simulink model "LQR_QRLsim"  (R2013b)
settings: Solver=ode45  StartTime=0.0  StopTime=Tsim_end  MaxStep=.1  RelTol=1e-3
values from neighbouring files (symbols this model uses):
  K = lqr(LQRA,LQRB,LQRQ,LQRR)    [LQRrunfile.m]
  LQRA = [zeros(8) eye(8) ... (first row only)    [LQRrunfile.m]
  LQRB = [zeros(10,4) ... (first row only)    [LQRrunfile.m]
  LQRC = eye(16)    [LQRrunfile.m]
  omega_n1_xL = 2*pi*.4    (= 2.51327412287)    [LQRrunfile.m]    (also in QRLrunfile.m = 25)
  omega_n2_xL = 2*pi*.4    (= 2.51327412287)    [LQRrunfile.m]
undefined symbols (not defined in the file or in its folder): sigbuilder_block, T0
libraries: CF3 x10, simulink x10, simulink_extras x2
settings Model: Creator=Nam  LastModifiedBy=Nam

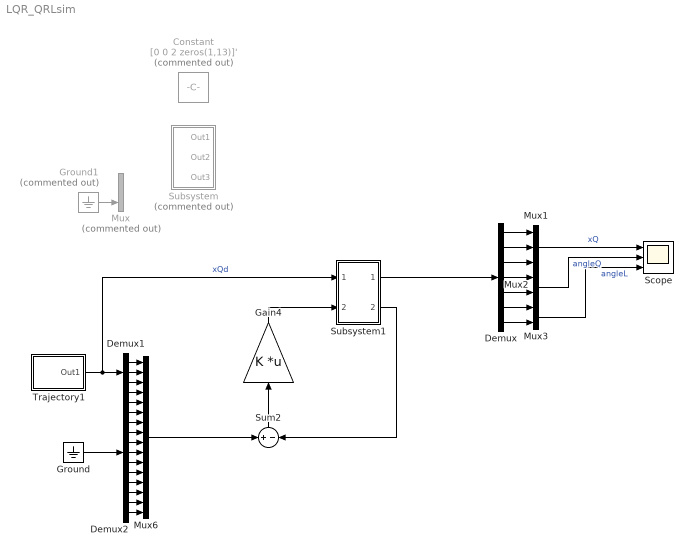
== system LQR_QRLsim ==
  Constant : Constant  Commented=on  Value=[0 0 2 zeros(1,13)]'
  Demux : Demux  Outputs=7
  Demux1 : Demux  Outputs=3
  Demux2 : Demux  Outputs=13
  Gain4 : Gain  Gain=K  Multiplication=Matrix(K*u)
  Ground : Ground
  Ground1 : Ground  Commented=on
  Mux : Mux  Commented=on  Inputs=2
  Mux1 : Mux  Inputs=3
  Mux2 : Mux  Inputs=2
  Mux3 : Mux  Inputs=2
  Mux6 : Mux  Inputs=16
  Scope : Scope  NumInputPorts=3
      settings: YMin=-5~-5~-5  YMax=5~5~5  SaveName=ScopeData9
  Subsystem : Subsystem  Commented=on
  Subsystem1 : Subsystem
  Sum2 : Sum  Inputs=+|-
  Trajectory1 : Subsystem
  wires:
  Sum2/1 -> Gain4/1
  Trajectory1/1(Out1) -> Subsystem1/1(In2), Demux1/1  "xQd"
  Demux1/1 -> Mux6/1
  Demux1/2 -> Mux6/2
  Demux1/3 -> Mux6/3
  Demux2/6 -> Mux6/9
  Demux2/11 -> Mux6/14
  Demux2/7 -> Mux6/10
  Demux2/10 -> Mux6/13
  Demux2/8 -> Mux6/11
  Demux2/12 -> Mux6/15
  Demux2/13 -> Mux6/16
  Demux2/5 -> Mux6/8
  Demux2/9 -> Mux6/12
  Demux2/4 -> Mux6/7
  Demux2/1 -> Mux6/4
  Demux2/2 -> Mux6/5
  Demux2/3 -> Mux6/6
  Ground/1 -> Demux2/1
  Gain4/1 -> Subsystem1/2(In1)
  Subsystem1/2(Out1) -> Sum2/2
  Ground1/1 -> Mux/2
  Mux6/1 -> Sum2/1
  Subsystem1/1(Out2) -> Demux/1
  Demux/2 -> Mux1/2
  Demux/1 -> Mux1/1
  Demux/3 -> Mux1/3
  Demux/4 -> Mux2/1
  Demux/5 -> Mux2/2
  Demux/6 -> Mux3/1
  Demux/7 -> Mux3/2
  Mux1/1 -> Scope/1  "xQ"
  Mux2/1 -> Scope/2  "angleQ"
  Mux3/1 -> Scope/3  "angleL"

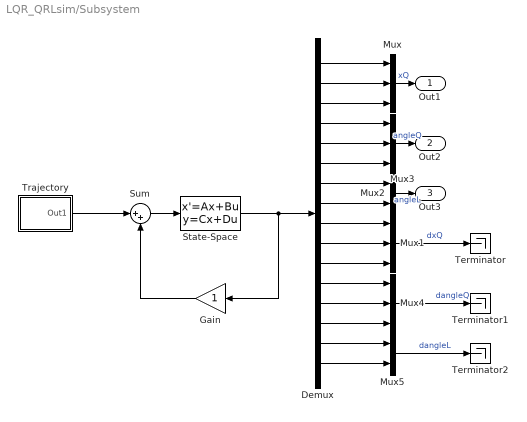
== system LQR_QRLsim/Subsystem ==
  Demux : Demux  Outputs=16
  Gain : Gain
  Mux{,1,3..4} (4 alike) : Mux  Inputs=3
  Mux2 : Mux  Inputs=2
  Mux5 : Mux  Inputs=2
  State-Space : StateSpace  A=LQRA  B=LQRB  C=LQRC  D=0  X0=0
  Sum : Sum  Inputs=|++
  Terminator : Terminator
  Terminator1 : Terminator
  Terminator2 : Terminator
  Trajectory : Subsystem
  Out1 : Outport
  Out2 : Outport  Port=2
  Out3 : Outport  Port=3
  wires:
  Trajectory/1(Out1) -> Sum/1
  Mux/1 -> Out1/1  "xQ"
  Mux3/1 -> Out2/1  "angleQ"
  Mux2/1 -> Out3/1  "angleL"
  Mux1/1 -> Terminator/1  "dxQ"
  Mux4/1 -> Terminator1/1  "dangleQ"
  Gain/1 -> Sum/2
  Demux/13 -> Mux4/2
  Sum/1 -> State-Space/1
  Mux5/1 -> Terminator2/1  "dangleL"
  Demux/16 -> Mux5/2
  Demux/14 -> Mux4/3
  Demux/12 -> Mux4/1
  Demux/15 -> Mux5/1
  Demux/8 -> Mux2/2
  Demux/7 -> Mux2/1
  Demux/10 -> Mux1/2
  Demux/5 -> Mux3/2
  Demux/6 -> Mux3/3
  Demux/9 -> Mux1/1
  Demux/11 -> Mux1/3
  Demux/4 -> Mux3/1
  Demux/1 -> Mux/1
  Demux/2 -> Mux/2
  Demux/3 -> Mux/3
  State-Space/1 -> Demux/1, Gain/1

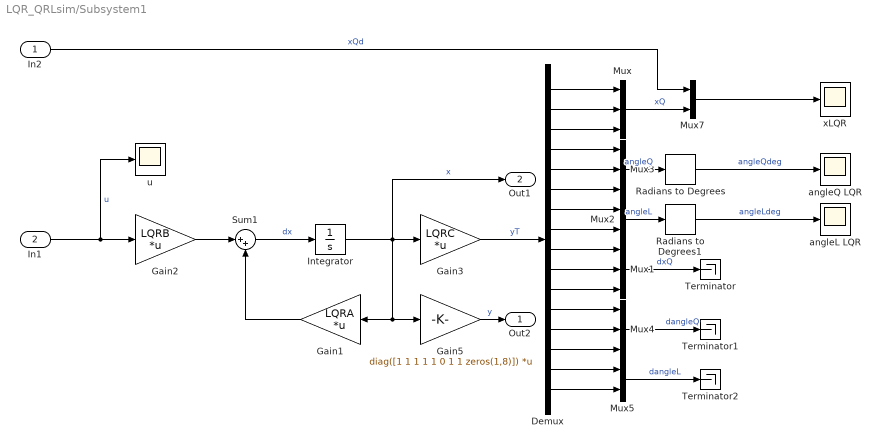
== system LQR_QRLsim/Subsystem1 ==
  In2 : Inport
  In1 : Inport  Port=2
  Demux : Demux  Outputs=16
  Gain1 : Gain  Gain=LQRA  Multiplication=Matrix(K*u)
  Gain2 : Gain  Gain=LQRB  Multiplication=Matrix(K*u)
  Gain3 : Gain  Gain=LQRC  Multiplication=Matrix(K*u)
  Gain5 : Gain  Gain=diag([1 1 1 1 1 0 1 1 zeros(1,8)])  Multiplication=Matrix(K*u)
  Integrator : Integrator
  Mux{,1,3..4} (4 alike) : Mux  Inputs=3
  Mux2 : Mux  Inputs=2
  Mux5 : Mux  Inputs=2
  Mux7 : Mux  Inputs=2
  Radians to Degrees : simulink_extras/Transformations/Radians to Degrees
  Radians to Degrees1 : simulink_extras/Transformations/Radians to Degrees
  Sum1 : Sum  Inputs=|++
  Terminator : Terminator
  Terminator1 : Terminator
  Terminator2 : Terminator
  angleL LQR : Scope
      settings: ShowLegends=on  TimeRange=25  YMin=-40  YMax=40  SaveName=ScopeData5
  angleQ LQR : Scope
      settings: ShowLegends=on  TimeRange=25  YMin=-40  YMax=40  SaveName=ScopeData4
  u : Scope
      settings: ShowLegends=on  SaveName=ScopeData8
  xLQR : Scope
      settings: ShowLegends=on  SaveName=ScopeData3
  Out2 : Outport
  Out1 : Outport  Port=2
  wires:
  Demux/3 -> Mux/3
  Demux/2 -> Mux/2
  Demux/1 -> Mux/1
  Demux/4 -> Mux3/1
  Demux/5 -> Mux3/2
  Demux/6 -> Mux3/3
  Demux/7 -> Mux2/1
  Demux/8 -> Mux2/2
  Demux/10 -> Mux1/2
  Demux/11 -> Mux1/3
  Demux/9 -> Mux1/1
  Demux/12 -> Mux4/1
  Demux/14 -> Mux4/3
  Demux/13 -> Mux4/2
  Demux/15 -> Mux5/1
  Demux/16 -> Mux5/2
  Mux1/1 -> Terminator/1  "dxQ"
  Mux4/1 -> Terminator1/1  "dangleQ"
  Mux5/1 -> Terminator2/1  "dangleL"
  Gain3/1 -> Demux/1  "yT"
  Mux/1 -> Mux7/2  "xQ"
  Mux3/1 -> Radians to Degrees/1  "angleQ"
  Mux2/1 -> Radians to Degrees1/1  "angleL"
  In1/1 -> u/1, Gain2/1  "u"
  Integrator/1 -> Out1/1, Gain3/1, Gain5/1, Gain1/1  "x"
  Sum1/1 -> Integrator/1  "dx"
  Gain1/1 -> Sum1/2
  Gain2/1 -> Sum1/1
  Mux7/1 -> xLQR/1
  Radians to Degrees/1 -> angleQ LQR/1  "angleQdeg"
  Radians to Degrees1/1 -> angleL LQR/1  "angleLdeg"
  In2/1 -> Mux7/1  "xQd"
  Gain5/1 -> Out2/1  "y"

== system LQR_QRLsim/Trajectory1 ==
  Circle : Subsystem  Commented=on
  Manual Switch : ManualSwitch  CurrentSetting=0
  Manual Switch1 : ManualSwitch  CurrentSetting=0
  Path : Subsystem
  Step : Subsystem
  Out1 : Outport
  wires:
  Manual Switch1/1 -> Out1/1  "xLd"
  Manual Switch/1 -> Manual Switch1/2
  Circle/1(Out3) -> Manual Switch1/1
  Path/1(Out3) -> Manual Switch/1
  Step/1(Out2) -> Manual Switch/2

== system LQR_QRLsim/Subsystem/Trajectory ==
  Circle : Subsystem
  Manual Switch : ManualSwitch
  Manual Switch1 : ManualSwitch  CurrentSetting=0
  Path : Subsystem
  Step : Subsystem
  Out1 : Outport
  wires:
  Step/1(Out2) -> Manual Switch/2
  Path/1(Out3) -> Manual Switch/1
  Circle/1(Out3) -> Manual Switch1/1
  Manual Switch/1 -> Manual Switch1/2
  Manual Switch1/1 -> Out1/1  "xLd"

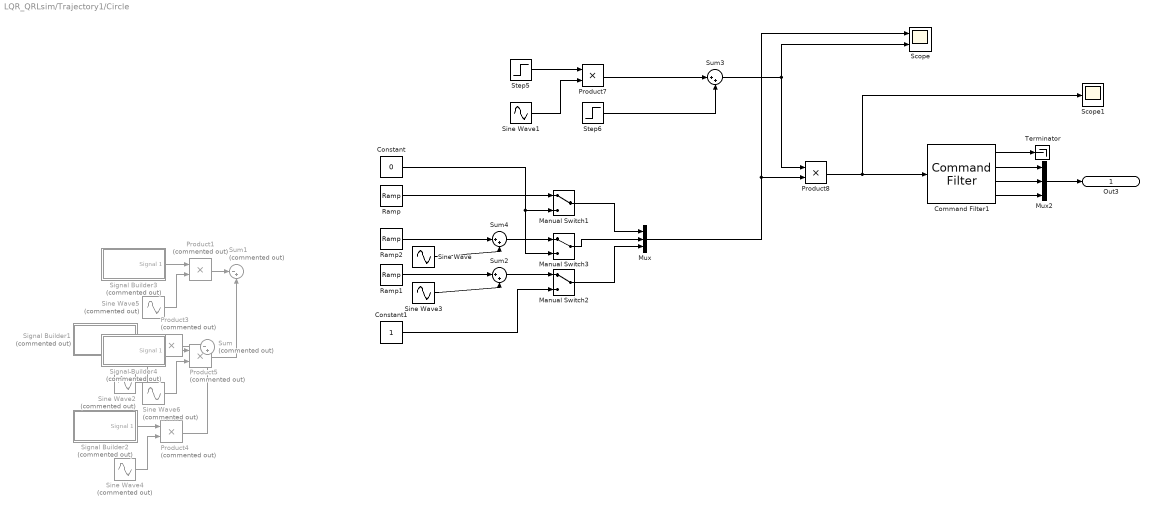
== system LQR_QRLsim/Trajectory1/Circle ==
  Command Filter1 : CF3/Command Filter  Integrator1_init=0  omega_n1=omega_n1_xL  omega_n2=omega_n2_xL  zeta=zeta_xL
  Constant : Constant  Value=0
  Constant1 : Constant
  Manual Switch1 : ManualSwitch
  Manual Switch2 : ManualSwitch
  Manual Switch3 : ManualSwitch
  Mux : Mux  Inputs=3
  Mux2 : Mux  Inputs=3
  Product{1,3..5} (4 alike) : Product  Commented=on
  Product7 : Product
  Product8 : Product
  Ramp : simulink/Sources/Ramp  slope=1/5  start=2  X0=0
  Ramp1 : simulink/Sources/Ramp  slope=0  start=0  X0=0
  Ramp2 : simulink/Sources/Ramp  slope=0  start=0  X0=0
  Scope : Scope  NumInputPorts=2
      settings: ShowLegends=on  YMin=-5~-5  YMax=5~5
  Scope1 : Scope
      settings: ShowLegends=on  YMin=-8  YMax=12  SaveName=ScopeData2
  Signal Builder1 : Subsystem  Tag=STV Subsys  Commented=on  LoadFcn=sigbuilder_block('load');  StartFcn=sigbuilder_block('start');  StopFcn=sigbuilder_block('stop');  ClipboardFcn=sigbuilder_block('clipboard');  mask(Sigbuilder block){}
      mask help: Simulink:masks:SigbuilderBlock_MD
      mask init:
      | if ~strcmp(get_param(bdroot(gcbh),'SimulationStatus'),'stopped') tuvar = sigbuilder_block('maskInit'); end
      settings: CopyFcn=sigbuilder_block('copy');  DeleteFcn=sigbuilder_block('delete');  ModelCloseFcn=sigbuilder_block('modelClose');  PreSaveFcn=sigbuilder_block('preSave');  PauseFcn=sigbuilder_block('pause');  ContinueFcn=sigbuilder_block('continue');  NameChangeFcn=sigbuilder_block('namechange');  OpenFcn=sigbuilder_block('open',[437.25 199.5 550.5 399.75 ]);  CloseFcn=sigbuilder_block('close');
      mask Display: plot(0, 0, 100, 100,[2, 2, 32, 32, 2], [68, 8, 8, 68, 68],[32, 2], [38, 38], [32, 19, 2],[53, 60, 44], [32, 17, 17, 2],[16, 16, 31, 31]);txt = getActiveGroup(gcbh);text(2, 100, txt,'verticalAlignment', 'top');
  Signal Builder2 : Subsystem  Tag=STV Subsys  Commented=on  LoadFcn=sigbuilder_block('load');  StartFcn=sigbuilder_block('start');  StopFcn=sigbuilder_block('stop');  ClipboardFcn=sigbuilder_block('clipboard');  mask(Sigbuilder block){}
      mask help: Simulink:masks:SigbuilderBlock_MD
      mask init:
      | if ~strcmp(get_param(bdroot(gcbh),'SimulationStatus'),'stopped') tuvar = sigbuilder_block('maskInit'); end
      settings: CopyFcn=sigbuilder_block('copy');  DeleteFcn=sigbuilder_block('delete');  ModelCloseFcn=sigbuilder_block('modelClose');  PreSaveFcn=sigbuilder_block('preSave');  PauseFcn=sigbuilder_block('pause');  ContinueFcn=sigbuilder_block('continue');  NameChangeFcn=sigbuilder_block('namechange');  OpenFcn=sigbuilder_block('open',[403.5 199.5 550.5 395.25 ]);  CloseFcn=sigbuilder_block('close');
      mask Display: plot(0, 0, 100, 100,[2, 2, 32, 32, 2], [68, 8, 8, 68, 68],[32, 2], [38, 38], [32, 19, 2],[53, 60, 44], [32, 17, 17, 2],[16, 16, 31, 31]);txt = getActiveGroup(gcbh);text(2, 100, txt,'verticalAlignment', 'top');
  Signal Builder3 : Subsystem  Tag=STV Subsys  Commented=on  LoadFcn=sigbuilder_block('load');  StartFcn=sigbuilder_block('start');  StopFcn=sigbuilder_block('stop');  ClipboardFcn=sigbuilder_block('clipboard');  mask(Sigbuilder block){}
      mask help: Simulink:masks:SigbuilderBlock_MD
      mask init:
      | if ~strcmp(get_param(bdroot(gcbh),'SimulationStatus'),'stopped') tuvar = sigbuilder_block('maskInit'); end
      settings: CopyFcn=sigbuilder_block('copy');  DeleteFcn=sigbuilder_block('delete');  ModelCloseFcn=sigbuilder_block('modelClose');  PreSaveFcn=sigbuilder_block('preSave');  PauseFcn=sigbuilder_block('pause');  ContinueFcn=sigbuilder_block('continue');  NameChangeFcn=sigbuilder_block('namechange');  OpenFcn=sigbuilder_block('open',[437.25 199.5 550.5 399.75 ]);  CloseFcn=sigbuilder_block('close');
      mask Display: plot(0, 0, 100, 100,[2, 2, 32, 32, 2], [68, 8, 8, 68, 68],[32, 2], [38, 38], [32, 19, 2],[53, 60, 44], [32, 17, 17, 2],[16, 16, 31, 31]);txt = getActiveGroup(gcbh);text(2, 100, txt,'verticalAlignment', 'top');
  Signal Builder4 : Subsystem  Tag=STV Subsys  Commented=on  LoadFcn=sigbuilder_block('load');  StartFcn=sigbuilder_block('start');  StopFcn=sigbuilder_block('stop');  ClipboardFcn=sigbuilder_block('clipboard');  mask(Sigbuilder block){}
      mask help: Simulink:masks:SigbuilderBlock_MD
      mask init:
      | if ~strcmp(get_param(bdroot(gcbh),'SimulationStatus'),'stopped') tuvar = sigbuilder_block('maskInit'); end
      settings: CopyFcn=sigbuilder_block('copy');  DeleteFcn=sigbuilder_block('delete');  ModelCloseFcn=sigbuilder_block('modelClose');  PreSaveFcn=sigbuilder_block('preSave');  PauseFcn=sigbuilder_block('pause');  ContinueFcn=sigbuilder_block('continue');  NameChangeFcn=sigbuilder_block('namechange');  OpenFcn=sigbuilder_block('open',[403.5 199.5 550.5 395.25 ]);  CloseFcn=sigbuilder_block('close');
      mask Display: plot(0, 0, 100, 100,[2, 2, 32, 32, 2], [68, 8, 8, 68, 68],[32, 2], [38, 38], [32, 19, 2],[53, 60, 44], [32, 17, 17, 2],[16, 16, 31, 31]);txt = getActiveGroup(gcbh);text(2, 100, txt,'verticalAlignment', 'top');
  Sine Wave : Sin  Amplitude=2.75  Frequency=2*pi/T0  Phase=-pi/2  SampleTime=0
  Sine Wave1 : Sin  Amplitude=0.5  Bias=0.5  Frequency=pi/(T0/2)  Phase=pi*1.5  SampleTime=0
  Sine Wave{2,4..6} (4 alike) : Sin  Commented=on  Amplitude=3  Frequency=2*pi/2.5  SampleTime=0
  Sine Wave3 : Sin  Frequency=2*pi/T0  SampleTime=0
  Step5 : Step  Time=(T0/2)  Before=1  After=0  SampleTime=0
  Step6 : Step  Time=(T0/2)  SampleTime=0
  Sum : Sum  Commented=on  Inputs=|-+
  Sum1 : Sum  Commented=on  Inputs=|-+
  Sum2 : Sum  Inputs=|++
  Sum3 : Sum  Inputs=|++
  Sum4 : Sum  Inputs=|++
  Terminator : Terminator
  Out3 : Outport
  wires:
  Constant/1 -> Manual Switch1/2, Manual Switch3/2
  Sine Wave3/1 -> Sum2/2
  Signal Builder1/1(Signal 1) -> Product3/1
  Sine Wave2/1 -> Product3/2
  Product3/1 -> Sum/1
  Signal Builder2/1(Signal 1) -> Product4/1
  Sine Wave4/1 -> Product4/2
  Product4/1 -> Sum/2
  Manual Switch3/1 -> Mux/2
  Manual Switch2/1 -> Mux/3
  Manual Switch1/1 -> Mux/1
  Mux/1 -> Product8/2, Scope/1
  Sine Wave1/1 -> Product7/2
  Step5/1 -> Product7/1
  Step6/1 -> Sum3/2
  Sum3/1 -> Product8/1, Scope/2
  Constant1/1 -> Manual Switch2/2
  Product7/1 -> Sum3/1
  Product8/1 -> Scope1/1, Command Filter1/1
  Signal Builder3/1(Signal 1) -> Product1/1
  Sine Wave5/1 -> Product1/2
  Product1/1 -> Sum1/1
  Signal Builder4/1(Signal 1) -> Product5/1
  Sine Wave6/1 -> Product5/2
  Product5/1 -> Sum1/2
  Ramp1/1 -> Sum2/1
  Ramp2/1 -> Sum4/1
  Sum4/1 -> Manual Switch3/1
  Sine Wave/1 -> Sum4/2
  Ramp/1 -> Manual Switch1/1
  Sum2/1 -> Manual Switch2/1
  Command Filter1/1 -> Terminator/1
  Command Filter1/3 -> Mux2/2
  Command Filter1/2 -> Mux2/1
  Command Filter1/4 -> Mux2/3
  Mux2/1 -> Out3/1

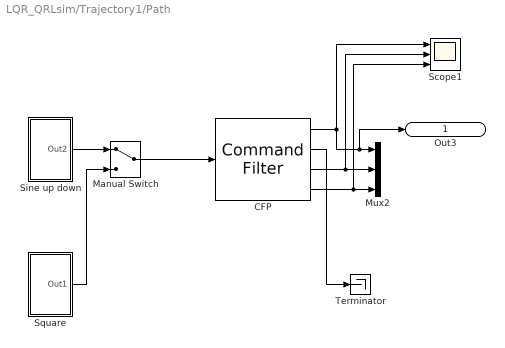
== system LQR_QRLsim/Trajectory1/Path ==
  CFP : CF3/Command Filter  Integrator1_init=0  omega_n1=omega_n1_xL*100  omega_n2=omega_n2_xL*50  zeta=zeta_xL
  Manual Switch : ManualSwitch
  Mux2 : Mux  Inputs=3
  Scope1 : Scope  NumInputPorts=3
      settings: TimeRange=25  YMin=-0.5~-0.8~-1.5  YMax=3.5~0.8~1.5  SaveName=ScopeData6
  Sine up down : Subsystem
  Square : Subsystem
  Terminator : Terminator
  Out3 : Outport
  wires:
  CFP/4 -> Scope1/3, Mux2/3
  CFP/3 -> Scope1/2, Mux2/2
  Manual Switch/1 -> CFP/1
  Square/1(Out1) -> Manual Switch/2
  Sine up down/1(Out2) -> Manual Switch/1
  CFP/1 -> Scope1/1, Out3/1, Mux2/1
  CFP/2 -> Terminator/1

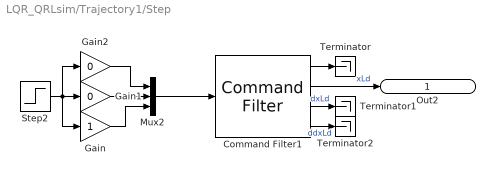
== system LQR_QRLsim/Trajectory1/Step ==
  Command Filter1 : CF3/Command Filter  Integrator1_init=0  omega_n1=2*pi*.75  omega_n2=2*pi*.75  zeta=.975
  Gain : Gain
  Gain1 : Gain  Gain=0
  Gain2 : Gain  Gain=0
  Mux2 : Mux  Inputs=3
  Step2 : Step  SampleTime=0
  Terminator : Terminator
  Terminator1 : Terminator
  Terminator2 : Terminator
  Out2 : Outport
  wires:
  Step2/1 -> Gain2/1, Gain/1, Gain1/1
  Mux2/1 -> Command Filter1/1
  Gain/1 -> Mux2/3
  Gain1/1 -> Mux2/2
  Gain2/1 -> Mux2/1
  Command Filter1/1 -> Terminator/1
  Command Filter1/2 -> Out2/1  "xLd"
  Command Filter1/3 -> Terminator1/1  "dxLd"
  Command Filter1/4 -> Terminator2/1  "ddxLd"

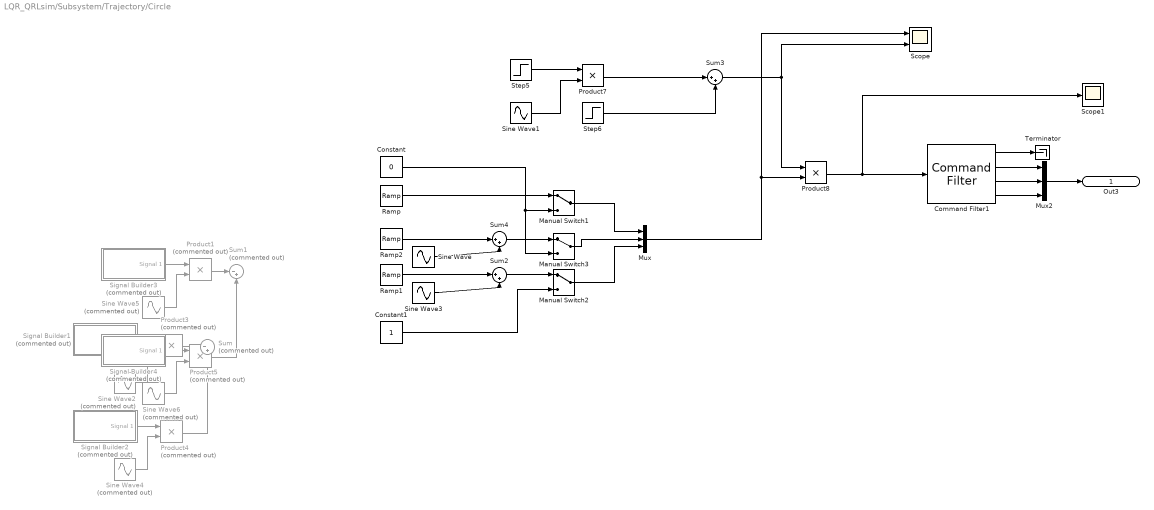
== system LQR_QRLsim/Subsystem/Trajectory/Circle ==
  Command Filter1 : CF3/Command Filter  Integrator1_init=0  omega_n1=omega_n1_xL  omega_n2=omega_n2_xL  zeta=zeta_xL
  Constant : Constant  Value=0
  Constant1 : Constant
  Manual Switch1 : ManualSwitch
  Manual Switch2 : ManualSwitch
  Manual Switch3 : ManualSwitch
  Mux : Mux  Inputs=3
  Mux2 : Mux  Inputs=3
  Product{1,3..5} (4 alike) : Product  Commented=on
  Product7 : Product
  Product8 : Product
  Ramp : simulink/Sources/Ramp  slope=1/5  start=2  X0=0
  Ramp1 : simulink/Sources/Ramp  slope=0  start=0  X0=0
  Ramp2 : simulink/Sources/Ramp  slope=0  start=0  X0=0
  Scope : Scope  NumInputPorts=2
      settings: ShowLegends=on  YMin=-5~-5  YMax=5~5
  Scope1 : Scope
      settings: ShowLegends=on  YMin=-8  YMax=12  SaveName=ScopeData2
  Signal Builder1 : Subsystem  Tag=STV Subsys  Commented=on  LoadFcn=sigbuilder_block('load');  StartFcn=sigbuilder_block('start');  StopFcn=sigbuilder_block('stop');  ClipboardFcn=sigbuilder_block('clipboard');  mask(Sigbuilder block){}
      mask help: Simulink:masks:SigbuilderBlock_MD
      mask init:
      | if ~strcmp(get_param(bdroot(gcbh),'SimulationStatus'),'stopped') tuvar = sigbuilder_block('maskInit'); end
      settings: CopyFcn=sigbuilder_block('copy');  DeleteFcn=sigbuilder_block('delete');  ModelCloseFcn=sigbuilder_block('modelClose');  PreSaveFcn=sigbuilder_block('preSave');  PauseFcn=sigbuilder_block('pause');  ContinueFcn=sigbuilder_block('continue');  NameChangeFcn=sigbuilder_block('namechange');  OpenFcn=sigbuilder_block('open',[437.25 199.5 550.5 399.75 ]);  CloseFcn=sigbuilder_block('close');
      mask Display: plot(0, 0, 100, 100,[2, 2, 32, 32, 2], [68, 8, 8, 68, 68],[32, 2], [38, 38], [32, 19, 2],[53, 60, 44], [32, 17, 17, 2],[16, 16, 31, 31]);txt = getActiveGroup(gcbh);text(2, 100, txt,'verticalAlignment', 'top');
  Signal Builder2 : Subsystem  Tag=STV Subsys  Commented=on  LoadFcn=sigbuilder_block('load');  StartFcn=sigbuilder_block('start');  StopFcn=sigbuilder_block('stop');  ClipboardFcn=sigbuilder_block('clipboard');  mask(Sigbuilder block){}
      mask help: Simulink:masks:SigbuilderBlock_MD
      mask init:
      | if ~strcmp(get_param(bdroot(gcbh),'SimulationStatus'),'stopped') tuvar = sigbuilder_block('maskInit'); end
      settings: CopyFcn=sigbuilder_block('copy');  DeleteFcn=sigbuilder_block('delete');  ModelCloseFcn=sigbuilder_block('modelClose');  PreSaveFcn=sigbuilder_block('preSave');  PauseFcn=sigbuilder_block('pause');  ContinueFcn=sigbuilder_block('continue');  NameChangeFcn=sigbuilder_block('namechange');  OpenFcn=sigbuilder_block('open',[403.5 199.5 550.5 395.25 ]);  CloseFcn=sigbuilder_block('close');
      mask Display: plot(0, 0, 100, 100,[2, 2, 32, 32, 2], [68, 8, 8, 68, 68],[32, 2], [38, 38], [32, 19, 2],[53, 60, 44], [32, 17, 17, 2],[16, 16, 31, 31]);txt = getActiveGroup(gcbh);text(2, 100, txt,'verticalAlignment', 'top');
  Signal Builder3 : Subsystem  Tag=STV Subsys  Commented=on  LoadFcn=sigbuilder_block('load');  StartFcn=sigbuilder_block('start');  StopFcn=sigbuilder_block('stop');  ClipboardFcn=sigbuilder_block('clipboard');  mask(Sigbuilder block){}
      mask help: Simulink:masks:SigbuilderBlock_MD
      mask init:
      | if ~strcmp(get_param(bdroot(gcbh),'SimulationStatus'),'stopped') tuvar = sigbuilder_block('maskInit'); end
      settings: CopyFcn=sigbuilder_block('copy');  DeleteFcn=sigbuilder_block('delete');  ModelCloseFcn=sigbuilder_block('modelClose');  PreSaveFcn=sigbuilder_block('preSave');  PauseFcn=sigbuilder_block('pause');  ContinueFcn=sigbuilder_block('continue');  NameChangeFcn=sigbuilder_block('namechange');  OpenFcn=sigbuilder_block('open',[437.25 199.5 550.5 399.75 ]);  CloseFcn=sigbuilder_block('close');
      mask Display: plot(0, 0, 100, 100,[2, 2, 32, 32, 2], [68, 8, 8, 68, 68],[32, 2], [38, 38], [32, 19, 2],[53, 60, 44], [32, 17, 17, 2],[16, 16, 31, 31]);txt = getActiveGroup(gcbh);text(2, 100, txt,'verticalAlignment', 'top');
  Signal Builder4 : Subsystem  Tag=STV Subsys  Commented=on  LoadFcn=sigbuilder_block('load');  StartFcn=sigbuilder_block('start');  StopFcn=sigbuilder_block('stop');  ClipboardFcn=sigbuilder_block('clipboard');  mask(Sigbuilder block){}
      mask help: Simulink:masks:SigbuilderBlock_MD
      mask init:
      | if ~strcmp(get_param(bdroot(gcbh),'SimulationStatus'),'stopped') tuvar = sigbuilder_block('maskInit'); end
      settings: CopyFcn=sigbuilder_block('copy');  DeleteFcn=sigbuilder_block('delete');  ModelCloseFcn=sigbuilder_block('modelClose');  PreSaveFcn=sigbuilder_block('preSave');  PauseFcn=sigbuilder_block('pause');  ContinueFcn=sigbuilder_block('continue');  NameChangeFcn=sigbuilder_block('namechange');  OpenFcn=sigbuilder_block('open',[403.5 199.5 550.5 395.25 ]);  CloseFcn=sigbuilder_block('close');
      mask Display: plot(0, 0, 100, 100,[2, 2, 32, 32, 2], [68, 8, 8, 68, 68],[32, 2], [38, 38], [32, 19, 2],[53, 60, 44], [32, 17, 17, 2],[16, 16, 31, 31]);txt = getActiveGroup(gcbh);text(2, 100, txt,'verticalAlignment', 'top');
  Sine Wave : Sin  Amplitude=2.75  Frequency=2*pi/T0  Phase=-pi/2  SampleTime=0
  Sine Wave1 : Sin  Amplitude=0.5  Bias=0.5  Frequency=pi/(T0/2)  Phase=pi*1.5  SampleTime=0
  Sine Wave{2,4..6} (4 alike) : Sin  Commented=on  Amplitude=3  Frequency=2*pi/2.5  SampleTime=0
  Sine Wave3 : Sin  Frequency=2*pi/T0  SampleTime=0
  Step5 : Step  Time=(T0/2)  Before=1  After=0  SampleTime=0
  Step6 : Step  Time=(T0/2)  SampleTime=0
  Sum : Sum  Commented=on  Inputs=|-+
  Sum1 : Sum  Commented=on  Inputs=|-+
  Sum2 : Sum  Inputs=|++
  Sum3 : Sum  Inputs=|++
  Sum4 : Sum  Inputs=|++
  Terminator : Terminator
  Out3 : Outport
  wires:
  Mux2/1 -> Out3/1
  Command Filter1/4 -> Mux2/3
  Command Filter1/2 -> Mux2/1
  Command Filter1/3 -> Mux2/2
  Command Filter1/1 -> Terminator/1
  Sum2/1 -> Manual Switch2/1
  Ramp/1 -> Manual Switch1/1
  Sine Wave/1 -> Sum4/2
  Sum4/1 -> Manual Switch3/1
  Ramp2/1 -> Sum4/1
  Ramp1/1 -> Sum2/1
  Product5/1 -> Sum1/2
  Sine Wave6/1 -> Product5/2
  Signal Builder4/1(Signal 1) -> Product5/1
  Product1/1 -> Sum1/1
  Sine Wave5/1 -> Product1/2
  Signal Builder3/1(Signal 1) -> Product1/1
  Product8/1 -> Command Filter1/1, Scope1/1
  Product7/1 -> Sum3/1
  Constant1/1 -> Manual Switch2/2
  Sum3/1 -> Scope/2, Product8/1
  Step6/1 -> Sum3/2
  Step5/1 -> Product7/1
  Sine Wave1/1 -> Product7/2
  Mux/1 -> Scope/1, Product8/2
  Manual Switch1/1 -> Mux/1
  Manual Switch2/1 -> Mux/3
  Manual Switch3/1 -> Mux/2
  Product4/1 -> Sum/2
  Sine Wave4/1 -> Product4/2
  Signal Builder2/1(Signal 1) -> Product4/1
  Product3/1 -> Sum/1
  Sine Wave2/1 -> Product3/2
  Signal Builder1/1(Signal 1) -> Product3/1
  Sine Wave3/1 -> Sum2/2
  Constant/1 -> Manual Switch3/2, Manual Switch1/2

== system LQR_QRLsim/Subsystem/Trajectory/Path ==
  CFP : CF3/Command Filter  Integrator1_init=0  omega_n1=omega_n1_xL*100  omega_n2=omega_n2_xL*50  zeta=zeta_xL
  Manual Switch : ManualSwitch  CurrentSetting=0
  Mux2 : Mux  Inputs=3
  Scope1 : Scope  NumInputPorts=3
      settings: TimeRange=25  YMin=-0.5~-0.8~-1.5  YMax=3.5~0.8~1.5  SaveName=ScopeData6
  Sine up down : Subsystem
  Square : Subsystem
  Terminator : Terminator
  Out3 : Outport
  wires:
  CFP/2 -> Terminator/1
  CFP/1 -> Mux2/1, Scope1/1
  Sine up down/1(Out2) -> Manual Switch/1
  Mux2/1 -> Out3/1
  Square/1(Out1) -> Manual Switch/2
  Manual Switch/1 -> CFP/1
  CFP/3 -> Mux2/2, Scope1/2
  CFP/4 -> Mux2/3, Scope1/3

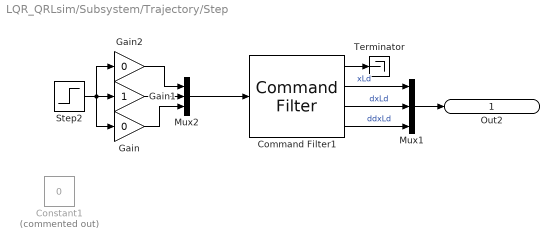
== system LQR_QRLsim/Subsystem/Trajectory/Step ==
  Command Filter1 : CF3/Command Filter  Integrator1_init=0  omega_n1=2*pi*.75  omega_n2=2*pi*.75  zeta=.975
  Constant1 : Constant  Commented=on  Value=0
  Gain : Gain  Gain=0
  Gain1 : Gain
  Gain2 : Gain  Gain=0
  Mux1 : Mux  Inputs=3
  Mux2 : Mux  Inputs=3
  Step2 : Step  SampleTime=0
  Terminator : Terminator
  Out2 : Outport
  wires:
  Mux1/1 -> Out2/1
  Command Filter1/3 -> Mux1/2  "dxLd"
  Command Filter1/2 -> Mux1/1  "xLd"
  Command Filter1/4 -> Mux1/3  "ddxLd"
  Command Filter1/1 -> Terminator/1
  Gain2/1 -> Mux2/1
  Gain1/1 -> Mux2/2
  Gain/1 -> Mux2/3
  Mux2/1 -> Command Filter1/1
  Step2/1 -> Gain1/1, Gain/1, Gain2/1

== system LQR_QRLsim/Trajectory1/Circle/Signal Builder1 ==
  Demux : Demux  Tag=STV Demux  Outputs=1
  FromWs : FromWorkspace  Tag=STV FromWs  VariableName=tuvar  SampleTime=0
      SigBuilderData=|
      | common.afterFinalStr = 'Extrapolate'
      | common.sampleTime = 0
      | dataSet.timeRange = [0 10]
      | dataSet.name = 'Group 1'
      | sbobj.Groups.Name = 'Group 1'
      | sbobj.Groups.Signals.Name = 'Signal 1'
      | sbobj.Groups.Signals.XData = [0 2.5 2.5 10]
      | sbobj.Groups.Signals.YData = [1 1 0 0]
  Signal 1 : Outport  Tag=STV Outport
  wires:
  Demux/1 -> Signal 1/1
  FromWs/1 -> Demux/1

== system LQR_QRLsim/Trajectory1/Circle/Signal Builder2 ==
  Demux : Demux  Tag=STV Demux  Outputs=1
  FromWs : FromWorkspace  Tag=STV FromWs  VariableName=tuvar  SampleTime=0
      SigBuilderData=|
      | common.afterFinalStr = 'Extrapolate'
      | common.sampleTime = 0
      | dataSet.timeRange = [0 10]
      | dataSet.name = 'Group 1'
      | sbobj.Groups.Name = 'Group 1'
      | sbobj.Groups.Signals.Name = 'Signal 1'
      | sbobj.Groups.Signals.XData = [0 2.5 2.5 5 5 10]
      | sbobj.Groups.Signals.YData = [0 0 1 1 0 0]
  Signal 1 : Outport  Tag=STV Outport
  wires:
  Demux/1 -> Signal 1/1
  FromWs/1 -> Demux/1

== system LQR_QRLsim/Trajectory1/Circle/Signal Builder3 ==
  Demux : Demux  Tag=STV Demux  Outputs=1
  FromWs : FromWorkspace  Tag=STV FromWs  VariableName=tuvar  SampleTime=0
      SigBuilderData=|
      | common.afterFinalStr = 'Extrapolate'
      | common.sampleTime = 0
      | dataSet.timeRange = [0 10]
      | dataSet.name = 'Group 1'
      | sbobj.Groups.Name = 'Group 1'
      | sbobj.Groups.Signals.Name = 'Signal 1'
      | sbobj.Groups.Signals.XData = [0 2.5 2.5 10]
      | sbobj.Groups.Signals.YData = [1 1 0 0]
  Signal 1 : Outport  Tag=STV Outport
  wires:
  FromWs/1 -> Demux/1
  Demux/1 -> Signal 1/1

== system LQR_QRLsim/Trajectory1/Circle/Signal Builder4 ==
  Demux : Demux  Tag=STV Demux  Outputs=1
  FromWs : FromWorkspace  Tag=STV FromWs  VariableName=tuvar  SampleTime=0
      SigBuilderData=|
      | common.afterFinalStr = 'Extrapolate'
      | common.sampleTime = 0
      | dataSet.timeRange = [0 10]
      | dataSet.name = 'Group 1'
      | sbobj.Groups.Name = 'Group 1'
      | sbobj.Groups.Signals.Name = 'Signal 1'
      | sbobj.Groups.Signals.XData = [0 2.5 2.5 5 5 10]
      | sbobj.Groups.Signals.YData = [0 0 1 1 0 0]
  Signal 1 : Outport  Tag=STV Outport
  wires:
  FromWs/1 -> Demux/1
  Demux/1 -> Signal 1/1

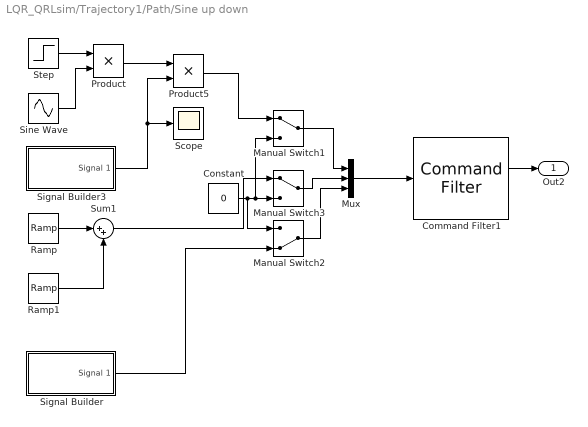
== system LQR_QRLsim/Trajectory1/Path/Sine up down ==
  Command Filter1 : CF3/Command Filter  Integrator1_init=0  omega_n1=omega_n1_xL  omega_n2=omega_n2_xL  zeta=zeta_xL
  Constant : Constant  Value=0
  Manual Switch1 : ManualSwitch
  Manual Switch2 : ManualSwitch  CurrentSetting=0
  Manual Switch3 : ManualSwitch
  Mux : Mux  Inputs=3
  Product : Product
  Product5 : Product
  Ramp : simulink/Sources/Ramp  slope=1/2  start=0  X0=0
  Ramp1 : simulink/Sources/Ramp  slope=-1/2  start=14  X0=0
  Scope : Scope
  Signal Builder : Subsystem  Tag=STV Subsys  LoadFcn=sigbuilder_block('load');  StartFcn=sigbuilder_block('start');  StopFcn=sigbuilder_block('stop');  ClipboardFcn=sigbuilder_block('clipboard');  mask(Sigbuilder block){}
      mask help: Simulink:masks:SigbuilderBlock_MD
      mask init:
      | if ~strcmp(get_param(bdroot(gcbh),'SimulationStatus'),'stopped') tuvar = sigbuilder_block('maskInit'); end
      settings: CopyFcn=sigbuilder_block('copy');  DeleteFcn=sigbuilder_block('delete');  ModelCloseFcn=sigbuilder_block('modelClose');  PreSaveFcn=sigbuilder_block('preSave');  PauseFcn=sigbuilder_block('pause');  ContinueFcn=sigbuilder_block('continue');  NameChangeFcn=sigbuilder_block('namechange');  OpenFcn=sigbuilder_block('open',[611.25 186.75 750 399.75 ]);  CloseFcn=sigbuilder_block('close');
      mask Display: plot(0, 0, 100, 100,[2, 2, 32, 32, 2], [68, 8, 8, 68, 68],[32, 2], [38, 38], [32, 19, 2],[53, 60, 44], [32, 17, 17, 2],[16, 16, 31, 31]);txt = getActiveGroup(gcbh);text(2, 100, txt,'verticalAlignment', 'top');
  Signal Builder3 : Subsystem  Tag=STV Subsys  LoadFcn=sigbuilder_block('load');  StartFcn=sigbuilder_block('start');  StopFcn=sigbuilder_block('stop');  ClipboardFcn=sigbuilder_block('clipboard');  mask(Sigbuilder block){}
      mask help: Simulink:masks:SigbuilderBlock_MD
      mask init:
      | if ~strcmp(get_param(bdroot(gcbh),'SimulationStatus'),'stopped') tuvar = sigbuilder_block('maskInit'); end
      settings: CopyFcn=sigbuilder_block('copy');  DeleteFcn=sigbuilder_block('delete');  ModelCloseFcn=sigbuilder_block('modelClose');  PreSaveFcn=sigbuilder_block('preSave');  PauseFcn=sigbuilder_block('pause');  ContinueFcn=sigbuilder_block('continue');  NameChangeFcn=sigbuilder_block('namechange');  OpenFcn=sigbuilder_block('open',[87.75 213.75 999 399.75 ]);  CloseFcn=sigbuilder_block('close');
      mask Display: plot(0, 0, 100, 100,[2, 2, 32, 32, 2], [68, 8, 8, 68, 68],[32, 2], [38, 38], [32, 19, 2],[53, 60, 44], [32, 17, 17, 2],[16, 16, 31, 31]);txt = getActiveGroup(gcbh);text(2, 100, txt,'verticalAlignment', 'top');
  Sine Wave : Sin  Amplitude=3  Frequency=2*pi/2.5  SampleTime=0
  Step : Step  Time=0  SampleTime=0
  Sum1 : Sum  Inputs=|++
  Out2 : Outport
  wires:
  Mux/1 -> Command Filter1/1
  Constant/1 -> Manual Switch3/2, Manual Switch1/2, Manual Switch2/1
  Manual Switch1/1 -> Mux/1
  Manual Switch2/1 -> Mux/3
  Ramp/1 -> Sum1/1
  Manual Switch3/1 -> Mux/2
  Step/1 -> Product/1
  Sine Wave/1 -> Product/2
  Product/1 -> Product5/1
  Product5/1 -> Manual Switch1/1
  Signal Builder3/1(Signal 1) -> Scope/1, Product5/2
  Ramp1/1 -> Sum1/2
  Sum1/1 -> Manual Switch3/1
  Signal Builder/1(Signal 1) -> Manual Switch2/2
  Command Filter1/2 -> Out2/1

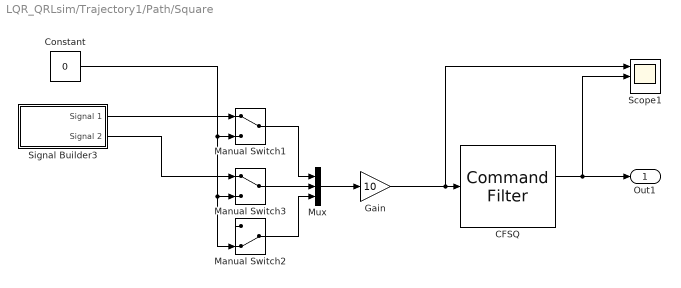
== system LQR_QRLsim/Trajectory1/Path/Square ==
  CFSQ : CF3/Command Filter  Integrator1_init=0  omega_n1=2*pi*1.2*0.5  omega_n2=2*pi*1*.5  zeta=zeta_xL
  Constant : Constant  Value=0
  Gain : Gain  Gain=10
  Manual Switch1 : ManualSwitch
  Manual Switch2 : ManualSwitch  CurrentSetting=0
  Manual Switch3 : ManualSwitch
  Mux : Mux  Inputs=3
  Scope1 : Scope  NumInputPorts=3
      settings: ShowLegends=on  TimeRange=15  YMin=0~0~-1  YMax=1~1~1  SaveName=ScopeData7
  Signal Builder3 : Subsystem  Tag=STV Subsys  LoadFcn=sigbuilder_block('load');  StartFcn=sigbuilder_block('start');  StopFcn=sigbuilder_block('stop');  ClipboardFcn=sigbuilder_block('clipboard');  mask(Sigbuilder block){}
      mask help: Simulink:masks:SigbuilderBlock_MD
      mask init:
      | if ~strcmp(get_param(bdroot(gcbh),'SimulationStatus'),'stopped') tuvar = sigbuilder_block('maskInit'); end
      settings: CopyFcn=sigbuilder_block('copy');  DeleteFcn=sigbuilder_block('delete');  ModelCloseFcn=sigbuilder_block('modelClose');  PreSaveFcn=sigbuilder_block('preSave');  PauseFcn=sigbuilder_block('pause');  ContinueFcn=sigbuilder_block('continue');  NameChangeFcn=sigbuilder_block('namechange');  OpenFcn=sigbuilder_block('open',[181.5 90.75 999 399.75 ]);  CloseFcn=sigbuilder_block('close');
      mask Display: plot(0, 0, 100, 100,[2, 2, 32, 32, 2], [68, 8, 8, 68, 68],[32, 2], [38, 38], [32, 19, 2],[53, 60, 44], [32, 17, 17, 2],[16, 16, 31, 31]);txt = getActiveGroup(gcbh);text(2, 100, txt,'verticalAlignment', 'top');
  Out1 : Outport
  wires:
  Constant/1 -> Manual Switch2/2, Manual Switch3/2, Manual Switch1/2
  Manual Switch1/1 -> Mux/1
  Manual Switch2/1 -> Mux/3
  Manual Switch3/1 -> Mux/2
  Mux/1 -> Gain/1
  CFSQ/2 -> Scope1/2, Out1/1
  Signal Builder3/1(Signal 1) -> Manual Switch1/1
  Signal Builder3/2(Signal 2) -> Manual Switch3/1
  Gain/1 -> Scope1/1, CFSQ/1

== system LQR_QRLsim/Subsystem/Trajectory/Circle/Signal Builder1 ==
  Demux : Demux  Tag=STV Demux  Outputs=1
  FromWs : FromWorkspace  Tag=STV FromWs  VariableName=tuvar  SampleTime=0
      SigBuilderData=|
      | common.afterFinalStr = 'Extrapolate'
      | common.sampleTime = 0
      | dataSet.timeRange = [0 10]
      | dataSet.name = 'Group 1'
      | sbobj.Groups.Name = 'Group 1'
      | sbobj.Groups.Signals.Name = 'Signal 1'
      | sbobj.Groups.Signals.XData = [0 2.5 2.5 10]
      | sbobj.Groups.Signals.YData = [1 1 0 0]
  Signal 1 : Outport  Tag=STV Outport
  wires:
  FromWs/1 -> Demux/1
  Demux/1 -> Signal 1/1

== system LQR_QRLsim/Subsystem/Trajectory/Circle/Signal Builder2 ==
  Demux : Demux  Tag=STV Demux  Outputs=1
  FromWs : FromWorkspace  Tag=STV FromWs  VariableName=tuvar  SampleTime=0
      SigBuilderData=|
      | common.afterFinalStr = 'Extrapolate'
      | common.sampleTime = 0
      | dataSet.timeRange = [0 10]
      | dataSet.name = 'Group 1'
      | sbobj.Groups.Name = 'Group 1'
      | sbobj.Groups.Signals.Name = 'Signal 1'
      | sbobj.Groups.Signals.XData = [0 2.5 2.5 5 5 10]
      | sbobj.Groups.Signals.YData = [0 0 1 1 0 0]
  Signal 1 : Outport  Tag=STV Outport
  wires:
  FromWs/1 -> Demux/1
  Demux/1 -> Signal 1/1

== system LQR_QRLsim/Subsystem/Trajectory/Circle/Signal Builder3 ==
  Demux : Demux  Tag=STV Demux  Outputs=1
  FromWs : FromWorkspace  Tag=STV FromWs  VariableName=tuvar  SampleTime=0
      SigBuilderData=|
      | common.afterFinalStr = 'Extrapolate'
      | common.sampleTime = 0
      | dataSet.timeRange = [0 10]
      | dataSet.name = 'Group 1'
      | sbobj.Groups.Name = 'Group 1'
      | sbobj.Groups.Signals.Name = 'Signal 1'
      | sbobj.Groups.Signals.XData = [0 2.5 2.5 10]
      | sbobj.Groups.Signals.YData = [1 1 0 0]
  Signal 1 : Outport  Tag=STV Outport
  wires:
  Demux/1 -> Signal 1/1
  FromWs/1 -> Demux/1

== system LQR_QRLsim/Subsystem/Trajectory/Circle/Signal Builder4 ==
  Demux : Demux  Tag=STV Demux  Outputs=1
  FromWs : FromWorkspace  Tag=STV FromWs  VariableName=tuvar  SampleTime=0
      SigBuilderData=|
      | common.afterFinalStr = 'Extrapolate'
      | common.sampleTime = 0
      | dataSet.timeRange = [0 10]
      | dataSet.name = 'Group 1'
      | sbobj.Groups.Name = 'Group 1'
      | sbobj.Groups.Signals.Name = 'Signal 1'
      | sbobj.Groups.Signals.XData = [0 2.5 2.5 5 5 10]
      | sbobj.Groups.Signals.YData = [0 0 1 1 0 0]
  Signal 1 : Outport  Tag=STV Outport
  wires:
  Demux/1 -> Signal 1/1
  FromWs/1 -> Demux/1

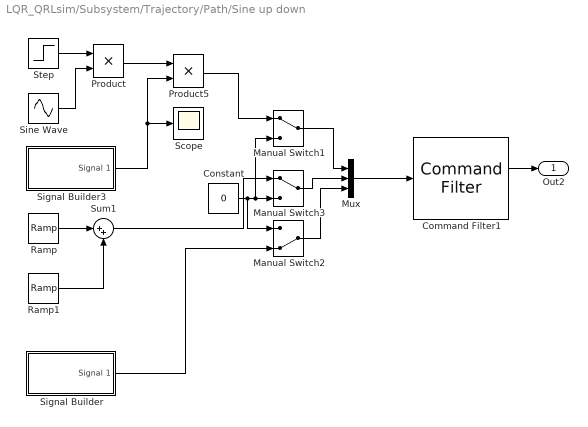
== system LQR_QRLsim/Subsystem/Trajectory/Path/Sine up down ==
  Command Filter1 : CF3/Command Filter  Integrator1_init=0  omega_n1=omega_n1_xL  omega_n2=omega_n2_xL  zeta=zeta_xL
  Constant : Constant  Value=0
  Manual Switch1 : ManualSwitch
  Manual Switch2 : ManualSwitch  CurrentSetting=0
  Manual Switch3 : ManualSwitch
  Mux : Mux  Inputs=3
  Product : Product
  Product5 : Product
  Ramp : simulink/Sources/Ramp  slope=1/2  start=0  X0=0
  Ramp1 : simulink/Sources/Ramp  slope=-1/2  start=14  X0=0
  Scope : Scope
  Signal Builder : Subsystem  Tag=STV Subsys  LoadFcn=sigbuilder_block('load');  StartFcn=sigbuilder_block('start');  StopFcn=sigbuilder_block('stop');  ClipboardFcn=sigbuilder_block('clipboard');  mask(Sigbuilder block){}
      mask help: Simulink:masks:SigbuilderBlock_MD
      mask init:
      | if ~strcmp(get_param(bdroot(gcbh),'SimulationStatus'),'stopped') tuvar = sigbuilder_block('maskInit'); end
      settings: CopyFcn=sigbuilder_block('copy');  DeleteFcn=sigbuilder_block('delete');  ModelCloseFcn=sigbuilder_block('modelClose');  PreSaveFcn=sigbuilder_block('preSave');  PauseFcn=sigbuilder_block('pause');  ContinueFcn=sigbuilder_block('continue');  NameChangeFcn=sigbuilder_block('namechange');  OpenFcn=sigbuilder_block('open',[611.25 186.75 750 399.75 ]);  CloseFcn=sigbuilder_block('close');
      mask Display: plot(0, 0, 100, 100,[2, 2, 32, 32, 2], [68, 8, 8, 68, 68],[32, 2], [38, 38], [32, 19, 2],[53, 60, 44], [32, 17, 17, 2],[16, 16, 31, 31]);txt = getActiveGroup(gcbh);text(2, 100, txt,'verticalAlignment', 'top');
  Signal Builder3 : Subsystem  Tag=STV Subsys  LoadFcn=sigbuilder_block('load');  StartFcn=sigbuilder_block('start');  StopFcn=sigbuilder_block('stop');  ClipboardFcn=sigbuilder_block('clipboard');  mask(Sigbuilder block){}
      mask help: Simulink:masks:SigbuilderBlock_MD
      mask init:
      | if ~strcmp(get_param(bdroot(gcbh),'SimulationStatus'),'stopped') tuvar = sigbuilder_block('maskInit'); end
      settings: CopyFcn=sigbuilder_block('copy');  DeleteFcn=sigbuilder_block('delete');  ModelCloseFcn=sigbuilder_block('modelClose');  PreSaveFcn=sigbuilder_block('preSave');  PauseFcn=sigbuilder_block('pause');  ContinueFcn=sigbuilder_block('continue');  NameChangeFcn=sigbuilder_block('namechange');  OpenFcn=sigbuilder_block('open',[87.75 213.75 999 399.75 ]);  CloseFcn=sigbuilder_block('close');
      mask Display: plot(0, 0, 100, 100,[2, 2, 32, 32, 2], [68, 8, 8, 68, 68],[32, 2], [38, 38], [32, 19, 2],[53, 60, 44], [32, 17, 17, 2],[16, 16, 31, 31]);txt = getActiveGroup(gcbh);text(2, 100, txt,'verticalAlignment', 'top');
  Sine Wave : Sin  Amplitude=3  Frequency=2*pi/2.5  SampleTime=0
  Step : Step  Time=0  SampleTime=0
  Sum1 : Sum  Inputs=|++
  Out2 : Outport
  wires:
  Command Filter1/2 -> Out2/1
  Signal Builder/1(Signal 1) -> Manual Switch2/2
  Sum1/1 -> Manual Switch3/1
  Ramp1/1 -> Sum1/2
  Signal Builder3/1(Signal 1) -> Product5/2, Scope/1
  Product5/1 -> Manual Switch1/1
  Product/1 -> Product5/1
  Sine Wave/1 -> Product/2
  Step/1 -> Product/1
  Manual Switch3/1 -> Mux/2
  Ramp/1 -> Sum1/1
  Manual Switch2/1 -> Mux/3
  Manual Switch1/1 -> Mux/1
  Constant/1 -> Manual Switch2/1, Manual Switch1/2, Manual Switch3/2
  Mux/1 -> Command Filter1/1

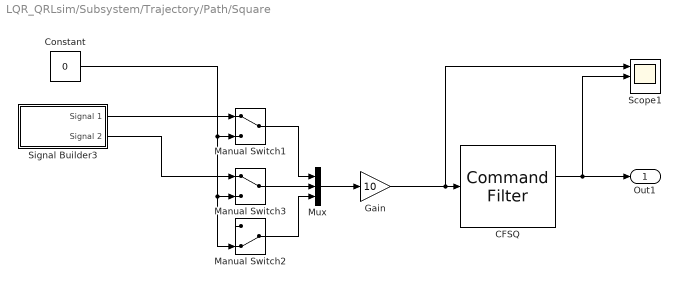
== system LQR_QRLsim/Subsystem/Trajectory/Path/Square ==
  CFSQ : CF3/Command Filter  Integrator1_init=0  omega_n1=2*pi*1.2*0.5  omega_n2=2*pi*1*.5  zeta=zeta_xL
  Constant : Constant  Value=0
  Gain : Gain  Gain=10
  Manual Switch1 : ManualSwitch
  Manual Switch2 : ManualSwitch  CurrentSetting=0
  Manual Switch3 : ManualSwitch
  Mux : Mux  Inputs=3
  Scope1 : Scope  NumInputPorts=3
      settings: ShowLegends=on  TimeRange=15  YMin=0~0~-1  YMax=1~1~1  SaveName=ScopeData7
  Signal Builder3 : Subsystem  Tag=STV Subsys  LoadFcn=sigbuilder_block('load');  StartFcn=sigbuilder_block('start');  StopFcn=sigbuilder_block('stop');  ClipboardFcn=sigbuilder_block('clipboard');  mask(Sigbuilder block){}
      mask help: Simulink:masks:SigbuilderBlock_MD
      mask init:
      | if ~strcmp(get_param(bdroot(gcbh),'SimulationStatus'),'stopped') tuvar = sigbuilder_block('maskInit'); end
      settings: CopyFcn=sigbuilder_block('copy');  DeleteFcn=sigbuilder_block('delete');  ModelCloseFcn=sigbuilder_block('modelClose');  PreSaveFcn=sigbuilder_block('preSave');  PauseFcn=sigbuilder_block('pause');  ContinueFcn=sigbuilder_block('continue');  NameChangeFcn=sigbuilder_block('namechange');  OpenFcn=sigbuilder_block('open',[181.5 90.75 999 399.75 ]);  CloseFcn=sigbuilder_block('close');
      mask Display: plot(0, 0, 100, 100,[2, 2, 32, 32, 2], [68, 8, 8, 68, 68],[32, 2], [38, 38], [32, 19, 2],[53, 60, 44], [32, 17, 17, 2],[16, 16, 31, 31]);txt = getActiveGroup(gcbh);text(2, 100, txt,'verticalAlignment', 'top');
  Out1 : Outport
  wires:
  Gain/1 -> CFSQ/1, Scope1/1
  Signal Builder3/2(Signal 2) -> Manual Switch3/1
  Signal Builder3/1(Signal 1) -> Manual Switch1/1
  CFSQ/2 -> Out1/1, Scope1/2
  Mux/1 -> Gain/1
  Manual Switch3/1 -> Mux/2
  Manual Switch2/1 -> Mux/3
  Manual Switch1/1 -> Mux/1
  Constant/1 -> Manual Switch1/2, Manual Switch3/2, Manual Switch2/2

== system LQR_QRLsim/Trajectory1/Path/Sine up down/Signal Builder ==
  Demux : Demux  Tag=STV Demux  Outputs=1
  FromWs : FromWorkspace  Tag=STV FromWs  VariableName=tuvar  SampleTime=0
      SigBuilderData=|
      | common.afterFinalStr = 'Extrapolate'
      | common.sampleTime = 0
      | dataSet.timeRange = [0 15]
      | dataSet.name = 'Group 1'
      | sbobj.Groups.Name = 'Group 1'
      | sbobj.Groups.Signals.Name = 'Signal 1'
      | sbobj.Groups.Signals.XData = [0 2 7.5 12.5 15]
      | sbobj.Groups.Signals.YData = [0 0 1 0 0]
      | sbobj.Groups.TimeRange = [0 15]
  Signal 1 : Outport  Tag=STV Outport
  wires:
  Demux/1 -> Signal 1/1
  FromWs/1 -> Demux/1

== system LQR_QRLsim/Trajectory1/Path/Sine up down/Signal Builder3 ==
  Demux : Demux  Tag=STV Demux  Outputs=1
  FromWs : FromWorkspace  Tag=STV FromWs  VariableName=tuvar  SampleTime=0
      SigBuilderData=|
      | common.afterFinalStr = 'Extrapolate'
      | common.sampleTime = 0
      | dataSet.timeRange = [0 20]
      | dataSet.name = 'Group 1'
      | sbobj.Groups.Name = 'Group 1'
      | sbobj.Groups.Signals.Name = 'Signal 1'
      | sbobj.Groups.Signals.XData = [0 4 10 14 20]
      | sbobj.Groups.Signals.YData = [0 1 1 0 0]
      | sbobj.Groups.TimeRange = [0 20]
  Signal 1 : Outport  Tag=STV Outport
  wires:
  Demux/1 -> Signal 1/1
  FromWs/1 -> Demux/1

== system LQR_QRLsim/Trajectory1/Path/Square/Signal Builder3 ==
  Demux : Demux  Tag=STV Demux  Outputs=2
  FromWs : FromWorkspace  Tag=STV FromWs  VariableName=tuvar  SampleTime=0
      SigBuilderData=|
      | common.afterFinalStr = 'Extrapolate'
      | common.sampleTime = 0
      | dataSet.timeRange = [0 20]
      | dataSet.name = 'Group 1'
      | sbobj.Groups.Name = 'Group 1'
      | sbobj.Groups.Signals(1).Name = 'Signal 1'
      | sbobj.Groups.Signals(1).XData = [0 1 5 9 13 20]
      | sbobj.Groups.Signals(1).YData = [0 0 1 1 0 0]
      | sbobj.Groups.Signals(2).Name = 'Signal 2'
      | sbobj.Groups.Signals(2).XData = [0 5 9 13 17 20]
      | sbobj.Groups.Signals(2).YData = [0 0 1 1 0 0]
      | sbobj.Groups.TimeRange = [0 20]
  Signal 1 : Outport  Tag=STV Outport
  Signal 2 : Outport  Tag=STV Outport  Port=2
  wires:
  Demux/1 -> Signal 1/1
  FromWs/1 -> Demux/1
  Demux/2 -> Signal 2/1

== system LQR_QRLsim/Subsystem/Trajectory/Path/Sine up down/Signal Builder ==
  Demux : Demux  Tag=STV Demux  Outputs=1
  FromWs : FromWorkspace  Tag=STV FromWs  VariableName=tuvar  SampleTime=0
      SigBuilderData=|
      | common.afterFinalStr = 'Extrapolate'
      | common.sampleTime = 0
      | dataSet.timeRange = [0 15]
      | dataSet.name = 'Group 1'
      | sbobj.Groups.Name = 'Group 1'
      | sbobj.Groups.Signals.Name = 'Signal 1'
      | sbobj.Groups.Signals.XData = [0 2 7.5 12.5 15]
      | sbobj.Groups.Signals.YData = [0 0 1 0 0]
      | sbobj.Groups.TimeRange = [0 15]
  Signal 1 : Outport  Tag=STV Outport
  wires:
  FromWs/1 -> Demux/1
  Demux/1 -> Signal 1/1

== system LQR_QRLsim/Subsystem/Trajectory/Path/Sine up down/Signal Builder3 ==
  Demux : Demux  Tag=STV Demux  Outputs=1
  FromWs : FromWorkspace  Tag=STV FromWs  VariableName=tuvar  SampleTime=0
      SigBuilderData=|
      | common.afterFinalStr = 'Extrapolate'
      | common.sampleTime = 0
      | dataSet.timeRange = [0 20]
      | dataSet.name = 'Group 1'
      | sbobj.Groups.Name = 'Group 1'
      | sbobj.Groups.Signals.Name = 'Signal 1'
      | sbobj.Groups.Signals.XData = [0 4 10 14 20]
      | sbobj.Groups.Signals.YData = [0 1 1 0 0]
      | sbobj.Groups.TimeRange = [0 20]
  Signal 1 : Outport  Tag=STV Outport
  wires:
  FromWs/1 -> Demux/1
  Demux/1 -> Signal 1/1

== system LQR_QRLsim/Subsystem/Trajectory/Path/Square/Signal Builder3 ==
  Demux : Demux  Tag=STV Demux  Outputs=2
  FromWs : FromWorkspace  Tag=STV FromWs  VariableName=tuvar  SampleTime=0
      SigBuilderData=|
      | common.afterFinalStr = 'Extrapolate'
      | common.sampleTime = 0
      | dataSet.timeRange = [0 20]
      | dataSet.name = 'Group 1'
      | sbobj.Groups.Name = 'Group 1'
      | sbobj.Groups.Signals(1).Name = 'Signal 1'
      | sbobj.Groups.Signals(1).XData = [0 1 5 9 13 20]
      | sbobj.Groups.Signals(1).YData = [0 0 1 1 0 0]
      | sbobj.Groups.Signals(2).Name = 'Signal 2'
      | sbobj.Groups.Signals(2).XData = [0 5 9 13 17 20]
      | sbobj.Groups.Signals(2).YData = [0 0 1 1 0 0]
      | sbobj.Groups.TimeRange = [0 20]
  Signal 1 : Outport  Tag=STV Outport
  Signal 2 : Outport  Tag=STV Outport  Port=2
  wires:
  Demux/2 -> Signal 2/1
  FromWs/1 -> Demux/1
  Demux/1 -> Signal 1/1
